simulink library "tensionLimitAoA_cl"  (R2022a)
settings: Solver=VariableStepAuto  StartTime=0.0  StopTime=10.0  RelTol=1e-3
undefined symbols (not defined in the file): pathCtrl
libraries: filteredPIDControllerAW_ul x1
settings Model: Creator=JohnJr  LastModifiedBy=lhill8
settings SolverCC: AlgebraicLoopSolver=TrustRegion
settings DebuggingCC: UnconnectedInputMsg=warning  UnconnectedOutputMsg=warning  UnconnectedLineMsg=warning  SFMachineParentedDataDiag=warning

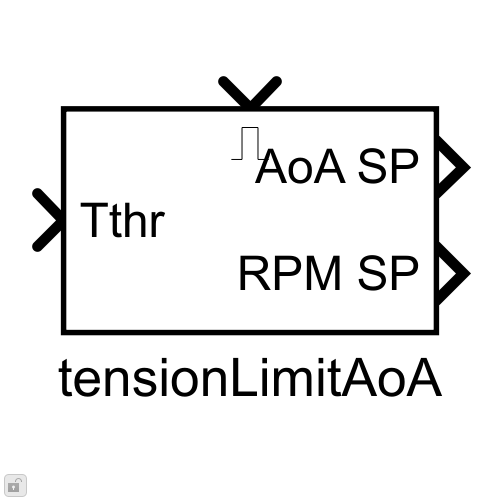
[thumbnail: Simulink's stored preview of the top-level diagram]
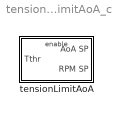
== system tensionLimitAoA_cl ==
  tensionLimitAoA : Subsystem

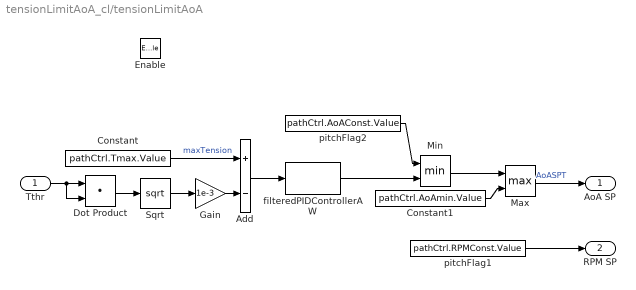
== system tensionLimitAoA_cl/tensionLimitAoA ==
  Tthr : Inport
  Enable : EnablePort
  Add : Sum  Inputs=+-
  Constant : Constant  Value=pathCtrl.Tmax.Value
  Constant1 : Constant  Value=pathCtrl.AoAmin.Value
  Dot Product : DotProduct  OutDataTypeStr=Inherit: Inherit via internal rule
  Gain : Gain  Gain=1e-3
  Max : MinMax  Function=max  Inputs=2
  Min : MinMax  Inputs=2
  Sqrt : Sqrt
  filteredPIDControllerAW : filteredPIDControllerAW_ul/filteredPIDControllerAW  kp=pathCtrl.alphaCtrl.kp.Value  ki=pathCtrl.alphaCtrl.ki.Value  kd=pathCtrl.alphaCtrl.kd.Value  tau=pathCtrl.alphaCtrl.tau.Value  cmax=pathCtrl.AoAConst.Value  cmin=pathCtrl.AoAmin.Value
  pitchFlag1 : Constant  Value=pathCtrl.RPMConst.Value
  pitchFlag2 : Constant  Value=pathCtrl.AoAConst.Value
  AoA SP : Outport
  RPM SP : Outport  Port=2
  wires:
  Tthr/1 -> Dot Product/2, Dot Product/1
  Dot Product/1 -> Sqrt/1
  Constant/1 -> Add/1  "maxTension"
  Sqrt/1 -> Gain/1
  Gain/1 -> Add/2
  Add/1 -> filteredPIDControllerAW/1
  pitchFlag2/1 -> Min/1
  Min/1 -> Max/1
  Max/1 -> AoA SP/1  "AoASPT"
  Constant1/1 -> Max/2
  filteredPIDControllerAW/1 -> Min/2
  pitchFlag1/1 -> RPM SP/1
